simulink model "driven_pendulum_case1"  (R2024b)
settings: Solver=VariableStepAuto  StartTime=0.0  StopTime=10.0  RelTol=1e-3
model workspace (MAT data in the model file):
  omegaB_0 = Simulink.Parameter
  omegaB_0.Value = 0
  omegaB_0.Complexity = 'real'
  omegaB_0.Dimensions = [1 1]
  omegaB_0.DataType = 'auto'
  thetaB_0 = 0.785398163397
settings Model: Creator=john_morris  LastModifiedBy=john_morris

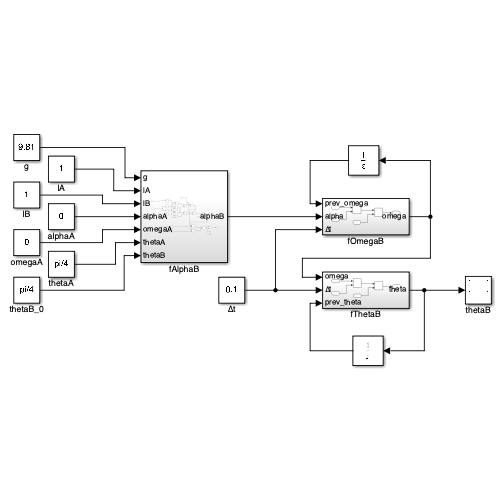
[thumbnail: Simulink's stored preview of the top-level diagram]
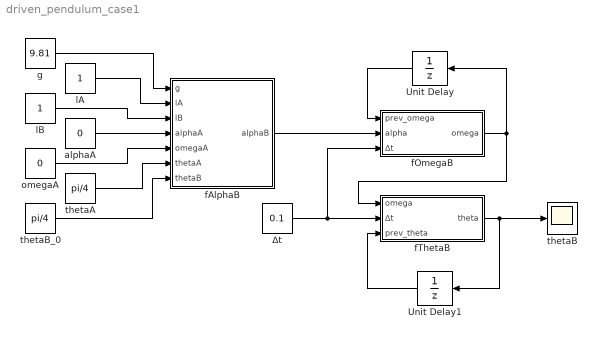
== system driven_pendulum_case1 ==
  Unit Delay : UnitDelay  InitialCondition=omegaB_0  SampleTime=-1  HasFrameUpgradeWarning=on
  Unit Delay1 : UnitDelay  InitialCondition=thetaB_0  SampleTime=-1  HasFrameUpgradeWarning=on
  alphaA : Constant  Value=0
  fAlphaB : Subsystem
  fOmegaB : Subsystem
  fThetaB : Subsystem
  g : Constant  Value=9.81
  lA : Constant
  lB : Constant
  omegaA : Constant  Value=0
  thetaA : Constant  Value=pi/4
  thetaB : Scope
  thetaB_0 : Constant  Value=pi/4
  ∆t : Constant  Value=0.1
  wires:
  thetaB_0/1 -> fAlphaB/7(thetaB)
  alphaA/1 -> fAlphaB/4(alphaA)
  thetaA/1 -> fAlphaB/6(thetaA)
  lA/1 -> fAlphaB/2(lA)
  g/1 -> fAlphaB/1(g)
  lB/1 -> fAlphaB/3(lB)
  fAlphaB/1(alphaB) -> fOmegaB/2(alpha)
  ∆t/1 -> fThetaB/2(∆t), fOmegaB/3(∆t)
  fOmegaB/1(omega) -> Unit Delay/1, fThetaB/1(omega)
  Unit Delay/1 -> fOmegaB/1(prev_omega)
  omegaA/1 -> fAlphaB/5(omegaA)
  Unit Delay1/1 -> fThetaB/3(prev_theta)
  fThetaB/1(theta) -> thetaB/1, Unit Delay1/1

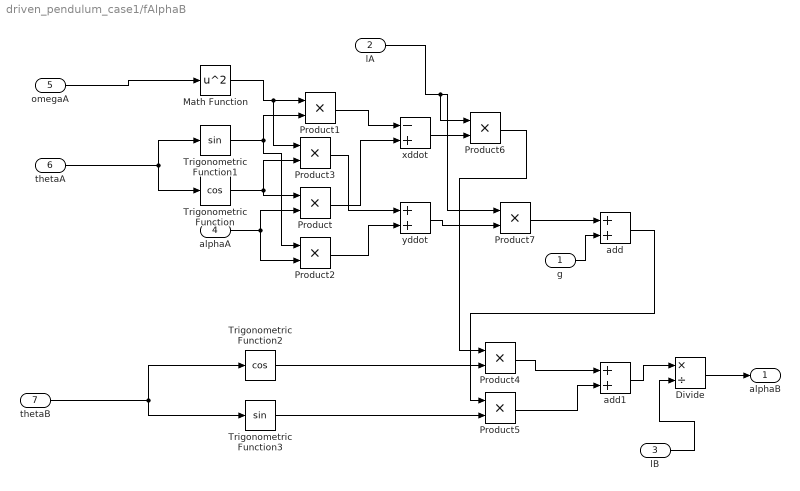
== system driven_pendulum_case1/fAlphaB ==
  g : Inport
  lA : Inport  Port=2
  lB : Inport  Port=3
  alphaA : Inport  Port=4
  omegaA : Inport  Port=5
  thetaA : Inport  Port=6
  thetaB : Inport  Port=7
  Divide : Product  Inputs=*/
  Math Function : Math  Operator=square
  Product{,1..7} (8 alike) : Product
  Trigonometric Function : Trigonometry  Operator=cos
  Trigonometric Function1 : Trigonometry
  Trigonometric Function2 : Trigonometry  Operator=cos
  Trigonometric Function3 : Trigonometry
  add : Sum
  add1 : Sum
  xddot : Sum  Inputs=-+
  yddot : Sum
  alphaB : Outport
  wires:
  thetaA/1 -> Trigonometric Function1/1, Trigonometric Function/1
  alphaA/1 -> Product2/2, Product/2
  Trigonometric Function/1 -> Product3/2, Product/1
  omegaA/1 -> Math Function/1
  Math Function/1 -> Product3/1, Product1/1
  Trigonometric Function1/1 -> Product2/1, Product1/2
  Product1/1 -> xddot/1
  Product/1 -> xddot/2
  Product2/1 -> yddot/2
  Product3/1 -> yddot/1
  thetaB/1 -> Trigonometric Function2/1, Trigonometric Function3/1
  Product6/1 -> Product4/1
  Trigonometric Function2/1 -> Product4/2
  yddot/1 -> Product7/2
  Trigonometric Function3/1 -> Product5/2
  g/1 -> add/2
  add/1 -> Product5/1
  Product4/1 -> add1/1
  Product5/1 -> add1/2
  add1/1 -> Divide/1
  lB/1 -> Divide/2
  Divide/1 -> alphaB/1
  xddot/1 -> Product6/2
  lA/1 -> Product7/1, Product6/1
  Product7/1 -> add/1

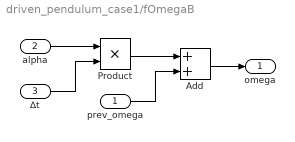
== system driven_pendulum_case1/fOmegaB ==
  prev_omega : Inport
  alpha : Inport  Port=2
  ∆t : Inport  Port=3
  Add : Sum
  Product : Product
  omega : Outport
  wires:
  alpha/1 -> Product/1
  ∆t/1 -> Product/2
  prev_omega/1 -> Add/2
  Product/1 -> Add/1
  Add/1 -> omega/1

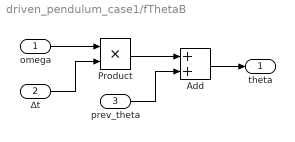
== system driven_pendulum_case1/fThetaB ==
  omega : Inport
  ∆t : Inport  Port=2
  prev_theta : Inport  Port=3
  Add : Sum
  Product : Product
  theta : Outport
  wires:
  omega/1 -> Product/1
  ∆t/1 -> Product/2
  prev_theta/1 -> Add/2
  Product/1 -> Add/1
  Add/1 -> theta/1
